simulink model "exemplo_prbs_input"  (Simulink 7.7)
settings: Solver=ode1  StartTime=0.0  StopTime=10.0  FixedStep=h  RelTol=1e-3
settings Model: Creator=jacoud  LastModifiedBy=jacoud
settings DataIOCC: SignalLoggingName=sigsOut
settings DebuggingCC: SaveWithParameterizedLinksMsg=none  SignalResolutionControl=TryResolveAllWithWarning  SolverPrmCheckMsg=none  MultiTaskDSMMsg=warning  MultiTaskCondExecSysMsg=none  StrictBusMsg=None
settings HardwareCC: TargetUnknown=on
settings RTWCC: IncludeERTFirstTime=on

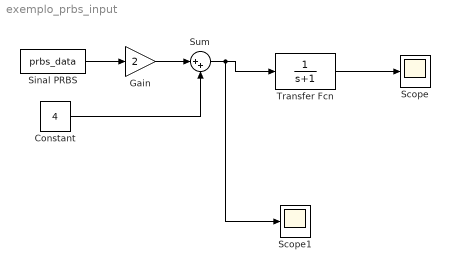
== system exemplo_prbs_input ==
  Constant : Constant  Value=4
  Gain : Gain  Gain=2  SaturateOnIntegerOverflow=on  OutDataTypeStr=Inherit: Same as input  ParamDataTypeStr=Inherit: Same as input
  Scope : Scope
  Scope1 : Scope
  Sinal PRBS : FromWorkspace  VariableName=prbs_data  SampleTime=0  OutputAfterFinalValue=Holding final value
  Sum : Sum  Inputs=|++  SaturateOnIntegerOverflow=on
  Transfer Fcn : TransferFcn  Denominator=[1 1]
  wires:
  Transfer Fcn/1 -> Scope/1
  Sinal PRBS/1 -> Gain/1
  Constant/1 -> Sum/2
  Gain/1 -> Sum/1
  Sum/1 -> Transfer Fcn/1, Scope1/1
